simulink model "PMSM_zhijieqidong"  (R2016a)
settings: Solver=ode45  StartTime=0.0  StopTime=1  MaxStep=1e-5  RelTol=1e-3
libraries: powerlib x5
settings Model: Creator=84360  LastModifiedBy=user

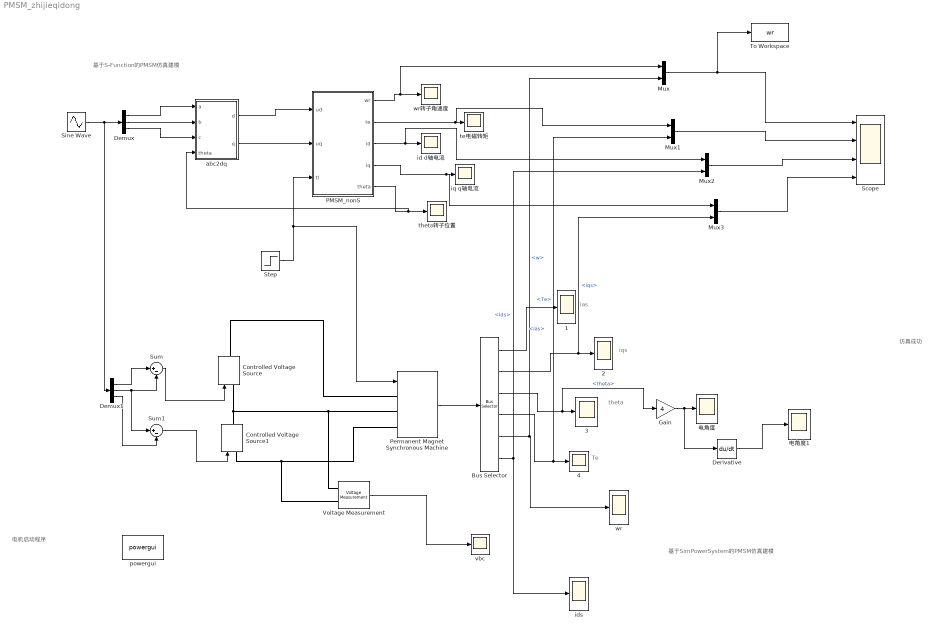
== system PMSM_zhijieqidong ==
  note: 仿真成功
  note: 基于S-Function的PMSM仿真建模
  note: 基于SimPowerSystem的PMSM仿真建模
  note: theta
  note: iqs
  note: ias
  note: Te
  note: 电机启动程序
  {1..4} (4 alike) : Scope
  Bus Selector : BusSelector  OutputSignals=ias,iqs,theta,Te,w,ids
  Controlled Voltage Source : powerlib/Electrical Sources/Controlled Voltage Source  Initialize=on  Source_Type=AC  Amplitude=0  Phase=0  Frequency=0  Measurements=None
  Controlled Voltage Source1 : powerlib/Electrical Sources/Controlled Voltage Source  Initialize=on  Source_Type=AC  Amplitude=0  Phase=0  Frequency=0  Measurements=None
  Demux : Demux  Outputs=3
  Demux1 : Demux  Outputs=3
  Derivative : Derivative
  Gain : Gain  Gain=4
  Mux{,1..3} (4 alike) : Mux  Inputs=2
  PMSM_nonS : Subsystem  mask{R=2.875, L=[8.5e-3 8.5e-3], psi_f=0.175, IFP=[0.8e-3 0 4], theta0=0, wr0=0, id0=0, iq0=0}
      mask prompts: R "Resistance R(ohm)"; L "Inductances[Ld(H) Lq(H)]:"; psi_f "Flux induced by magnets(Wb)"; IFP "inertia,friction factor and pairs of poles[J(kg.m^2 mu_f(N.m.s) p() ]"; theta0 "theta"
  Permanent Magnet Synchronous Machine : powerlib/Machines/Permanent Magnet Synchronous Machine  NbPhases=3  FluxDistribution=Sinusoidal  RotorType=Salient-pole  MechanicalLoad=Torque Tm  PresetModel=No  ShowDetailedParameters=on  MeasurementBus=on  Resistance=2.8750  Inductance=8.5e-3  dqInductances=[8.5e-3,8.5e-3]  La=0.000395  MachineConstant=Flux linkage established by magnets (V.s)  Flux=0.175  VoltageCst=126.966  TorqueCst=1.05  Flat=120  Mechanical=[0.0008 0.001 4 0]  PolePairs=4  InitialConditions=[0,0, 0,0]  InitialConditions5ph=[0 0 0 0 0 0]  TsPowergui=0  TsBlock=-1  RefAngle=Aligned with phase A axis (original Park)
  Scope : Scope  NumInputPorts=4
  Sine Wave : Sin  Amplitude=220*sqrt(2)  Frequency=20*pi  Phase=[0 -2*pi/3 2*pi/3]-[-pi/2 -pi/2 -pi/2]  SampleTime=0
  Step : Step  Time=0.3  Before=1  After=5  SampleTime=0
  Sum : Sum  Inputs=|+-
  Sum1 : Sum  Inputs=|+-
  To Workspace : ToWorkspace  VariableName=wr  SaveFormat=Timeseries  SampleTime=-1
  Voltage Measurement : powerlib/Measurements/Voltage Measurement  PhasorSimulation=off  OutputType=Complex  PSBequivalent=0
  abc2dq : Subsystem
  id d轴电流 : Scope
  ids : Scope
  iq q轴电流 : Scope
  powergui : powerlib/powergui  Priority=1  SimulationMode=Continuous  SolverType=Tustin/Backward Euler (TBE)  SampleTime=50e-6  frequency=60  SPID=off  DisableSnubberDevices=off  DisableRonSwitches=off  DisableVfSwitches=off  SwTol=0  DisplayEquations=off  Interpol=off  ExternalGateDelay=off  methode=off  Ts=10  FunctionMessages=off  echomessages=off  HookPort=off  EnableUseOfTLC=off  x0status=blocks  frequencyindice=0  Pbase=100e6  ErrMax=1e-4  Iterations=50  UnitsV=kV  UnitsW=MW  buscounter=0  RestoreLinks=warning  ResistiveCurrentMeasurement=off  Frange=[0:2:500]  Ylog=off  Xlog=on  ShowGrid=off  save=off  variable=ZData  structure=0  ZoomFFT=off  StartTime=0.0  cycles=1  DisplayStyle=1  fundamental=60  FreqAxis=off  MaxFrequency=1000  frequencyindicesteady=1  RmsSteady=1  display=off
  te电磁转矩 : Scope
  theta转子位置 : Scope
  vbc : Scope
  wr : Scope
  wr转子角速度 : Scope
  电角度 : Scope
  电角度1 : Scope
  wires:
  Step/1 -> Permanent Magnet Synchronous Machine/1, PMSM_nonS/3(tl)
  PMSM_nonS/3(id) -> Mux2/1, id d轴电流/1
  PMSM_nonS/4(iq) -> Mux3/1, iq q轴电流/1
  PMSM_nonS/1(wr) -> Mux/1, wr转子角速度/1
  PMSM_nonS/2(te) -> Mux1/1, te电磁转矩/1
  Demux/1 -> abc2dq/1(a)
  Demux/2 -> abc2dq/2(b)
  Demux/3 -> abc2dq/3(c)
  PMSM_nonS/5(theta) -> abc2dq/4(theta), theta转子位置/1
  abc2dq/1(d) -> PMSM_nonS/1(ud)
  abc2dq/2(q) -> PMSM_nonS/2(uq)
  Sine Wave/1 -> Demux1/1, Demux/1
  Permanent Magnet Synchronous Machine/1 -> Bus Selector/1
  Sum/1 -> Controlled Voltage Source/1
  Sum1/1 -> Controlled Voltage Source1/1
  Voltage Measurement/1 -> vbc/1
  Bus Selector/1 -> 1/1  "<ias>"
  Bus Selector/2 -> Mux3/2, 2/1  "<iqs>"
  Bus Selector/3 -> Gain/1, 3/1  "<theta>"
  Bus Selector/4 -> Mux1/2, 4/1  "<Te>"
  Bus Selector/5 -> Mux/2, wr/1  "<w>"
  Bus Selector/6 -> ids/1, Mux2/2  "<ids>"
  Demux1/1 -> Sum/1
  Demux1/2 -> Sum/2, Sum1/1
  Demux1/3 -> Sum1/2
  Mux/1 -> To Workspace/1, Scope/1
  Mux1/1 -> Scope/2
  Mux2/1 -> Scope/3
  Mux3/1 -> Scope/4
  Gain/1 -> Derivative/1, 电角度/1
  Derivative/1 -> 电角度1/1
  connections:
  Permanent Magnet Synchronous Machine/LConn2 -- Voltage Measurement/LConn1 -- Controlled Voltage Source1/RConn1 -- Controlled Voltage Source/LConn1
  Permanent Magnet Synchronous Machine/LConn3 -- Controlled Voltage Source1/LConn1 -- Voltage Measurement/LConn2
  Controlled Voltage Source/RConn1 -- Permanent Magnet Synchronous Machine/LConn1

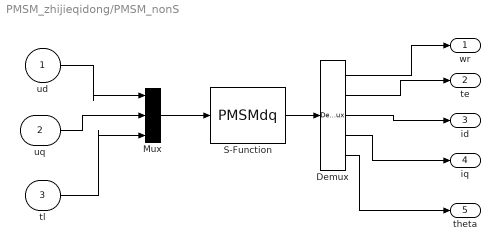
== system PMSM_zhijieqidong/PMSM_nonS ==
  ud : Inport
  uq : Inport  Port=2
  tl : Inport  Port=3
  Demux : Demux  Outputs=5
  Mux : Mux  Inputs=3
  S-Function : S-Function  FunctionName=PMSMdq  Parameters=[L R psi_f IFP(3) IFP(1) IFP(2)],[id0,iq0,wr0,theta0]  SFunctionDeploymentMode=off  EnableBusSupport=off  mask{R=2.875, L=[8.5e-3 8.5e-3], psi_f=0.175, IFP=[0.8e-3 0 4], theta0=0, wr0=0, id0=0, iq0=0}
      mask prompts: R "Resistance R(ohm):"; L "Inductances[Ld(H) Lq(H)]:"; psi_f "Flux induced by magnets(Wb):"; IFP "Inertia,friction factor and pairs of poles[J(kg.m^2)  mu_f(N.m.s)  p() ]:"
  wr : Outport
  te : Outport  Port=2
  id : Outport  Port=3
  iq : Outport  Port=4
  theta : Outport  Port=5
  wires:
  Demux/3 -> id/1
  uq/1 -> Mux/2
  ud/1 -> Mux/1
  Demux/4 -> iq/1
  Demux/2 -> te/1
  Mux/1 -> S-Function/1
  S-Function/1 -> Demux/1
  Demux/1 -> wr/1
  Demux/5 -> theta/1
  tl/1 -> Mux/3

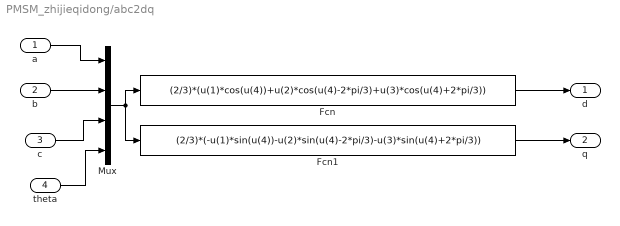
== system PMSM_zhijieqidong/abc2dq ==
  a : Inport
  b : Inport  Port=2
  c : Inport  Port=3
  theta : Inport  Port=4
  Fcn : Fcn  Expr=(2/3)*(u(1)*cos(u(4))+u(2)*cos(u(4)-2*pi/3)+u(3)*cos(u(4)+2*pi/3))
  Fcn1 : Fcn  Expr=(2/3)*(-u(1)*sin(u(4))-u(2)*sin(u(4)-2*pi/3)-u(3)*sin(u(4)+2*pi/3))
  Mux : Mux
  d : Outport
  q : Outport  Port=2
  wires:
  Mux/1 -> Fcn1/1, Fcn/1
  Fcn1/1 -> q/1
  c/1 -> Mux/3
  b/1 -> Mux/2
  a/1 -> Mux/1
  theta/1 -> Mux/4
  Fcn/1 -> d/1
